simulink model "rev0BB"  (R2014b)
settings: Solver=FixedStepDiscrete  SolverMode=SingleTasking  StartTime=0  StopTime=12000*basePer  RelTol=1e-3
StartFcn:
  | clc;
StopFcn:
  | disp('');
values from neighbouring files (symbols this model uses):
  baseFreq = overSampleFreq/overSample    (= 62.5)    [rev0BB_setup.m]    (also in rev0BB_startup.m = 31.25)
  basePer = 1/baseFreq    (= 0.016)    [rev0BB_setup.m]    (also in rev0BB_startup.m = 0.032)
  cbTol = int16(5)    [rev0BB_setup.m]    (also in rev0BB_startup.m)
  cef_note_len = uint16(length(cef_note))    [rev0BB_setup.m]    (also in rev0BB_startup.m)
  cr_int_amp = 2^-4    (= 0.0625)    [rev0BB_setup.m]
  cr_int_preamp = 2^-8    (= 0.00390625)    [rev0BB_setup.m]
  cr_pre_amp = 1    [rev0BB_setup.m]
  cr_smooth_amp = 2^-4    (= 0.0625)    [rev0BB_setup.m]
  cr_smooth_num = (1/cr_smooth_samples).*ones(1, cr_smooth_samples)    [rev0BB_setup.m]
  cr_smooth_second_denom = [1, -0.30]    [rev0BB_setup.m]
  D_128 = [ 1,  8,  2,  4, 16, 32, 64]    [golay.m]    (also in rev0BB_setup.m; rev0BB_startup.m = D_128 .* 4)
  dataDelay = length(cat(1, xCTRL_PRE_adj, guard, startWord)) + 1 + 187    [rev0BB_setup.m]    (also in rev0BB_startup.m = length(cat(1, xCTRL_PRE_adj, guard, startWord)) + 1)
  dataLen = 4096    [rev0BB_setup.m]    (also in rev0BB_startup.m)
  expDomain = 3.3    [rev0BB_setup.m]    (also in rev0BB_startup.m)
  expectedPer = int16(128*expectedWidth)    [rev0BB_setup.m]    (also in rev0BB_startup.m)
  expectedWidth = int16(1)    [rev0BB_setup.m]    (also in rev0BB_startup.m = int16(4))
  expResolution = 2^-7    (= 0.0078125)    [rev0BB_setup.m]    (also in rev0BB_startup.m)
  expTol = .1    (= 0.1)    [rev0BB_setup.m]    (also in rev0BB_startup.m)
  freqOffsetFactor = 0.001    [rev0BB_setup.m]
  guardInt = int16(4)    [rev0BB_setup.m]    (also in rev0BB_startup.m)
  guardTol = int16(5)    [rev0BB_setup.m]    (also in rev0BB_startup.m)
  invertedTol = int16(8)    [rev0BB_setup.m]    (also in rev0BB_startup.m)
  lineWidth = 60    [rev0BB_setup.m]    (also in rev0BB_startup.m)
  mult_pipeline = 3    [rev0BB_setup.m]
  overSamplePer = 1/overSampleFreq    (= 0.004)    [rev0BB_setup.m]    (also in rev0BB_startup.m = 0.008)
  rcRxFilt = [0.0136862302916632 -1.07255950749522e-17 -0.0189771276893529 -0.0291239876115654 -0.0188755211158258 0.0106361356824736 0.0424635782726055 0.0519988855587596 0.023305426798367 -0.0360582703762239 -0.092415015279578 -0.100052449159764 -0.0262868760771072 0.126203946316784 0.313718534732932 0.467989970028836 0.527600531456874 0.467989970028836 0.313718534732932 0.126203946316784 -0.0262868760771072 ...(+235 chars)    [rev0BB_setup.m]
  regular_pipeline = 1    [rev0BB_setup.m]
  smooth_num = (1).*(1/smooth_samples).*ones(1, smooth_samples)    [rev0BB_setup.m]
  smooth_scale = 0.0003    [rev0BB_setup.m]
  smooth_second_denom = [1, -0.95]    [rev0BB_setup.m]
  tol = int16(15)    [rev0BB_setup.m]    (also in rev0BB_startup.m)
  trigger = 60    [rev0BB_setup.m]    (also in rev0BB_startup.m)
  W_128 = [-1, -1, -1, -1, +1, -1, -1]    [golay.m]    (also in rev0BB_setup.m; rev0BB_startup.m)
  wordLen = int16(8)    [rev0BB_setup.m]    (also in rev0BB_startup.m)
undefined symbols (not defined in the file or in its folder): i, idealX
libraries: helperLib x11, golayLib x7, simulink x5, commdigbbndpm3 x4, dsparch4 x2, dspmlti4 x2, commfilt2 x2, commchan3 x1, commsink2 x1, commrflib2 x1, dspsigops x1, hdlsllib x1
settings Model: FPTRunName=FPA_Reference  Creator=cyarp  LastModifiedBy=cyarp
settings DataIOCC: SaveOutput=off  SignalLogging=off  SaveTime=off
settings OptimizationCC: BlockReduction=off  ConditionallyExecuteInputs=off  InlineParams=on  SimCompilerOptimization=On
settings DebuggingCC: AlgebraicLoopMsg=error  SingleTaskRateTransMsg=error
settings HardwareCC: ProdHWDeviceType=ASIC/FPGA->ASIC/FPGA  TargetBitPerLong=64  TargetBitPerPointer=64  TargetLongLongMode=on  TargetIntDivRoundTo=Zero  TargetEndianess=LittleEndian  TargetWordSize=64  TargetHWDeviceType=MATLAB Host  ProdEqTarget=off

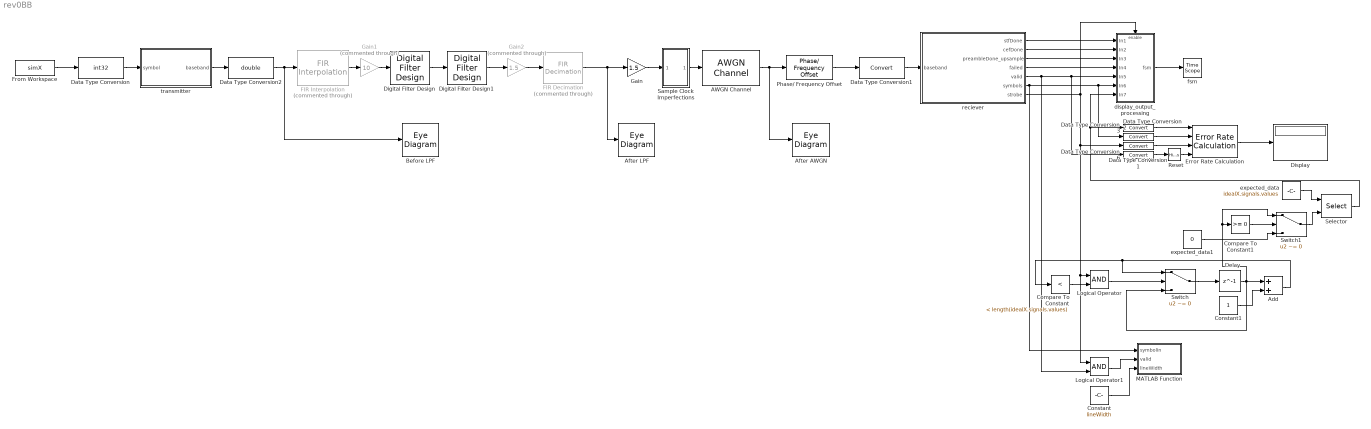
== system rev0BB ==
  AWGN Channel : commchan3/AWGN Channel  InputProcessing=Columns as channels (frame based)  seed=67  noiseMode="Signal to noise ratio  (Eb/No)"  EbNodB=awgnEbN0  EsNodB=10  SNRdB=10  bitsPerSym=1  Ps=1  Tsym=basePer*4  variance=1
  Add : Sum
  After AWGN : EyeDiagram
  After LPF : EyeDiagram
  Before LPF : EyeDiagram
  Compare To Constant : simulink/Logic and Bit Operations/Compare To Constant  relop=<  const=length(idealX.signals.values)  OutDataTypeStr=boolean
  Compare To Constant1 : simulink/Logic and Bit Operations/Compare To Constant  relop=>=  const=0  OutDataTypeStr=boolean
  Constant : Constant  Value=lineWidth
  Constant1 : Constant
  Data Type Conversion{1,1..3,6} (5 alike) : DataTypeConversion
  Data Type Conversion : DataTypeConversion  OutDataTypeStr=int32  RndMeth=Nearest
  Data Type Conversion2 : DataTypeConversion  OutDataTypeStr=double  RndMeth=Nearest
  Delay : Delay  DelayLength=1  InitialCondition=-dataDelay
  Digital Filter Design : dsparch4/Digital Filter Design  mwdsp_browser_bugfix_var=off
  Digital Filter Design1 : dsparch4/Digital Filter Design  mwdsp_browser_bugfix_var=off
  Display : Display
  Error Rate Calculation : commsink2/Error Rate Calculation  N=0  st_delay=0  cp_mode=Select samples from port  subframe=[]  PMode=Port  WsName=ErrorVec  RsMode2=on  stop=off  numErr=100  maxBits=1e6
  FIR Decimation : dspmlti4/FIR Decimation  Commented=through  h=fir1(35,0.4)  D=16  filtStruct=Direct form  framing=Enforce single-rate processing  inputOffset=0  outputBufInitCond=0  InputProcessing=Columns as channels (frame based)  firstCoeffDataTypeStr=Inherit: Same word length as input  firstCoeffLastDataTypeStr=Inherit: Same word length as input  firstCoeffMin=[]  firstCoeffMax=[]  outputDataTypeStr=Inherit: Same as accumulator  outputLastDataTypeStr=Inherit: Same as accumulator  outputMin=[]  outputMax=[]  roundingMode=Floor  overflowMode=off  FilterSource=Specify via dialog  FilterObject=Hm_firdecim
      settings: allowOverrides=off
  FIR Interpolation : dspmlti4/FIR Interpolation  Commented=through  h=fir1(15,1/4)  L=16  framing=Enforce single-rate processing  outputBufInitCond=0  InputProcessing=Columns as channels (frame based)  firstCoeffDataTypeStr=Inherit: Same word length as input  firstCoeffLastDataTypeStr=Inherit: Same word length as input  firstCoeffMin=[]  firstCoeffMax=[]  outputDataTypeStr=Inherit: Same as accumulator  outputLastDataTypeStr=Inherit: Same as accumulator  outputMin=[]  outputMax=[]  roundingMode=Floor  overflowMode=off  FilterSource=Specify via dialog  FilterObject=Hm_firinterp
  From Workspace : FromWorkspace  VariableName=simX  SampleTime=basePer*1  Interpolate=off  OutputAfterFinalValue=Setting to zero
  Gain : Gain  Gain=1.5
  Gain1 : Gain  Commented=through  Gain=10
  Gain2 : Gain  Commented=through  Gain=1.5
  Logical Operator : Logic  AllPortsSameDT=off  OutDataTypeStr=boolean
  Logical Operator1 : Logic  AllPortsSameDT=off  OutDataTypeStr=boolean
  MATLAB Function : MATLAB Function  TreatAsAtomicUnit=on
  Phase/ Frequency Offset : commrflib2/Phase// Frequency Offset  phaseOffset=180  freqPort=off  freqOffset=freqOffsetFactor*baseFreq
  Reset : HitCross  HitCrossingOffset=0.5  HitCrossingDirection=rising
  Sample Clock Imperfections : Subsystem
  Selector : Selector  IndexMode=Zero-based  InputPortWidth=length(idealX.signals.values)  IndexOptions=Index vector (port)  Indices=[1 3]
  Switch : Switch  Criteria=u2 ~= 0
  Switch1 : Switch  Criteria=u2 ~= 0
  display_output_processing : Subsystem
  expected_data : Constant  Value=idealX.signals.values
  expected_data1 : Constant  Value=0
  fsm : TimeScope  DefaultConfigurationName=spbscopes.TimeScopeBlockCfg
  reciever : Subsystem
  transmitter : Subsystem
  wires:
  Data Type Conversion1/1 -> reciever/1(baseband)
  Data Type Conversion/1 -> transmitter/1(symbol)
  transmitter/1(baseband) -> Data Type Conversion2/1
  From Workspace/1 -> Data Type Conversion/1
  Digital Filter Design1/1 -> Gain2/1
  Gain/1 -> Sample Clock Imperfections/1(In1)
  Digital Filter Design/1 -> Digital Filter Design1/1
  Sample Clock Imperfections/1(Out1) -> AWGN Channel/1
  AWGN Channel/1 -> After AWGN/1, Phase/ Frequency Offset/1
  Phase/ Frequency Offset/1 -> Data Type Conversion1/1
  reciever/1(stfDone) -> display_output_processing/1(In1)
  reciever/2(cefDone) -> display_output_processing/2(In2)
  reciever/3(preambleDone_upsample) -> display_output_processing/3(In3)
  reciever/4(failed) -> display_output_processing/4(In4)
  reciever/5(valid) -> Logical Operator1/2, Data Type Conversion6/1, display_output_processing/5(In5)
  Selector/1 -> Data Type Conversion3/1, display_output_processing/7(In7)
  display_output_processing/1(fsm) -> fsm/1
  Error Rate Calculation/1 -> Display/1
  Data Type Conversion6/1 -> Reset/1
  Reset/1 -> Error Rate Calculation/4
  Data Type Conversion1/1 -> Error Rate Calculation/3
  Data Type Conversion2/1 -> Error Rate Calculation/2
  Data Type Conversion3/1 -> Error Rate Calculation/1
  expected_data/1 -> Selector/1
  Constant1/1 -> Add/2
  Add/1 -> Switch/1, Compare To Constant/1
  Switch/1 -> Delay/1
  Compare To Constant/1 -> Logical Operator/2
  Logical Operator/1 -> Switch/2
  Delay/1 -> Switch1/1, Compare To Constant1/1, Switch/3, Add/1
  Switch1/1 -> Selector/2
  Compare To Constant1/1 -> Switch1/2
  expected_data1/1 -> Switch1/3
  reciever/7(strobe) -> display_output_processing/Enable, Logical Operator1/1, Logical Operator/1, Data Type Conversion1/1
  reciever/6(symbols) -> MATLAB Function/1(symbolIn), display_output_processing/6(In6), Data Type Conversion2/1
  Constant/1 -> MATLAB Function/3(lineWidth)
  Logical Operator1/1 -> MATLAB Function/2(valid)
  FIR Interpolation/1 -> Gain1/1
  Data Type Conversion2/1 -> FIR Interpolation/1, Before LPF/1
  Gain1/1 -> Digital Filter Design/1
  FIR Decimation/1 -> After LPF/1, Gain/1
  Gain2/1 -> FIR Decimation/1

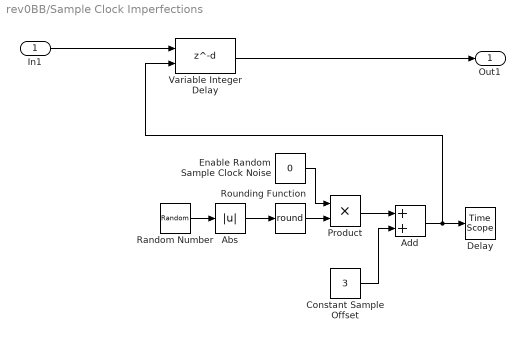
== system rev0BB/Sample Clock Imperfections ==
  In1 : Inport
  Abs : Abs
  Add : Sum
  Constant Sample Offset : Constant  Value=3
  Delay : TimeScope  DefaultConfigurationName=spbscopes.TimeScopeBlockCfg
  Enable Random Sample Clock Noise : Constant  Value=0
  Product : Product
  Random Number : RandomNumber  Variance=.5  SampleTime=overSamplePer
  Rounding Function : Rounding  Operator=round
  Variable Integer Delay : Delay  DelayLengthSource=Input port
      settings: InputPortMap=u0,p1
  Out1 : Outport
  wires:
  Abs/1 -> Rounding Function/1
  Random Number/1 -> Abs/1
  Add/1 -> Delay/1, Variable Integer Delay/2
  Enable Random Sample Clock Noise/1 -> Product/1
  Constant Sample Offset/1 -> Add/2
  Rounding Function/1 -> Product/2
  Product/1 -> Add/1
  In1/1 -> Variable Integer Delay/1
  Variable Integer Delay/1 -> Out1/1

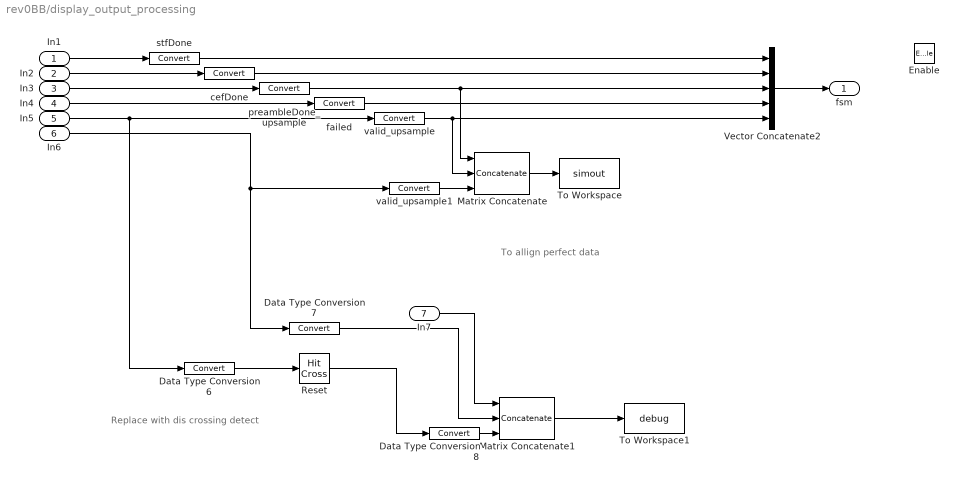
== system rev0BB/display_output_processing ==
  note: To allign perfect data
  note: Replace with dis crossing detect
  In1 : Inport
  In2 : Inport  Port=2
  In3 : Inport  Port=3
  In4 : Inport  Port=4
  In5 : Inport  Port=5
  In6 : Inport  Port=6
  In7 : Inport  Port=7
  Enable : EnablePort
  Data Type Conversion6 : DataTypeConversion
  Data Type Conversion7 : DataTypeConversion
  Data Type Conversion8 : DataTypeConversion
  Matrix Concatenate : Concatenate  NumInputs=3  Mode=Multidimensional array  ConcatenateDimension=2
  Matrix Concatenate1 : Concatenate  NumInputs=3  Mode=Multidimensional array  ConcatenateDimension=2
  Reset : HitCross  HitCrossingOffset=0.5  HitCrossingDirection=rising
  To Workspace : ToWorkspace  VariableName=simout  SampleTime=-1
      settings: Save2DSignal=2-D array (concatenate along first dimension)
  To Workspace1 : ToWorkspace  VariableName=debug  SampleTime=-1
      settings: Save2DSignal=2-D array (concatenate along first dimension)
  Vector Concatenate2 : Concatenate  NumInputs=5  Mode=Multidimensional array  ConcatenateDimension=2
  cefDone : DataTypeConversion
  failed : DataTypeConversion
  preambleDone_upsample : DataTypeConversion
  stfDone : DataTypeConversion
  valid_upsample : DataTypeConversion
  valid_upsample1 : DataTypeConversion
  fsm : Outport
  wires:
  Vector Concatenate2/1 -> fsm/1
  Matrix Concatenate/1 -> To Workspace/1
  stfDone/1 -> Vector Concatenate2/1
  cefDone/1 -> Vector Concatenate2/2
  preambleDone_upsample/1 -> Matrix Concatenate/1, Vector Concatenate2/3
  failed/1 -> Vector Concatenate2/4
  Data Type Conversion6/1 -> Reset/1
  In7/1 -> Matrix Concatenate1/1
  Matrix Concatenate1/1 -> To Workspace1/1
  Data Type Conversion8/1 -> Matrix Concatenate1/3
  Data Type Conversion7/1 -> Matrix Concatenate1/2
  Reset/1 -> Data Type Conversion8/1
  In1/1 -> stfDone/1
  In2/1 -> cefDone/1
  In3/1 -> preambleDone_upsample/1
  In4/1 -> failed/1
  valid_upsample/1 -> Matrix Concatenate/2, Vector Concatenate2/5
  valid_upsample1/1 -> Matrix Concatenate/3
  In5/1 -> Data Type Conversion6/1, valid_upsample/1
  In6/1 -> Data Type Conversion7/1, valid_upsample1/1

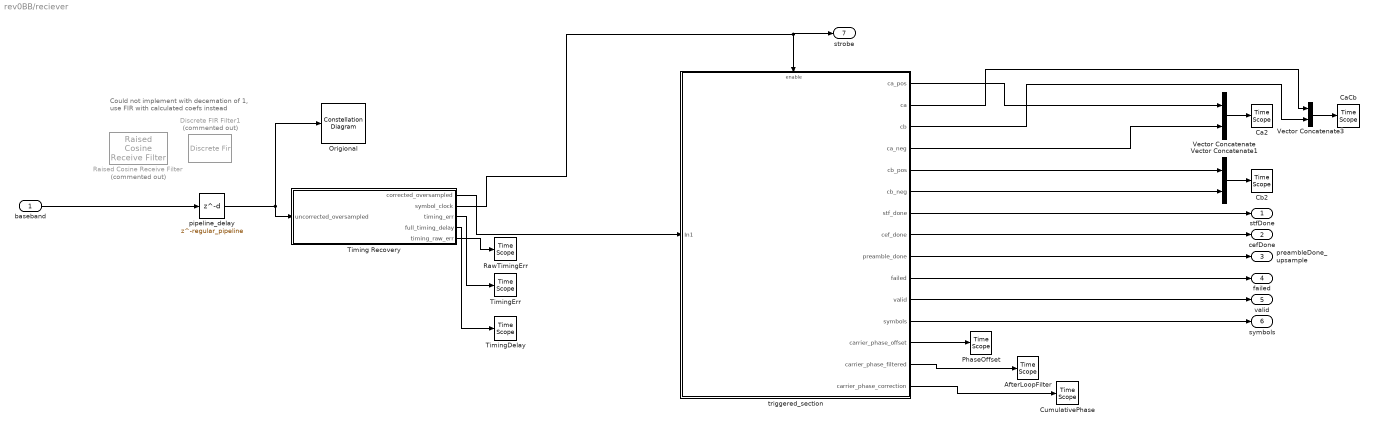
== system rev0BB/reciever ==
  note: Could not implement with decemation
      | of 1, use FIR with calculated coefs instead
  baseband : Inport  OutDataTypeStr=fixdt(1,14,11)  SampleTime=overSamplePer
  AfterLoopFilter : TimeScope  DefaultConfigurationName=spbscopes.TimeScopeBlockCfg
  Ca2 : TimeScope  DefaultConfigurationName=spbscopes.TimeScopeBlockCfg
  CaCb : TimeScope  DefaultConfigurationName=spbscopes.TimeScopeBlockCfg
  Cb2 : TimeScope  DefaultConfigurationName=spbscopes.TimeScopeBlockCfg
  CumulativePhase : TimeScope  DefaultConfigurationName=spbscopes.TimeScopeBlockCfg
  Discrete FIR Filter1 : DiscreteFir  Commented=on  Coefficients=rcRxFilt
  Origional : ConstellationDiagram
  PhaseOffset : TimeScope  DefaultConfigurationName=spbscopes.TimeScopeBlockCfg
  Raised Cosine Receive Filter : commfilt2/Raised Cosine Receive Filter  Commented=on  filtType=Normal  N=4  filtSpan=16  currentFiltSpan=16  D=(16)/2  R=.2  sampMode=Mute  saveAsFlag=0  rateMode=Downsampling  downFactor=1  downOffset=0  framing=Allow multirate processing  checkGain=Normalized  filterGain=1  checkCoeff=on  variableName=rcRxFilt  launchFVT=on  roundingMode=Floor  overflowMode=off
  RawTimingErr : TimeScope  DefaultConfigurationName=spbscopes.TimeScopeBlockCfg
  Timing Recovery : Subsystem
  TimingDelay : TimeScope  DefaultConfigurationName=spbscopes.TimeScopeBlockCfg
  TimingErr : TimeScope  DefaultConfigurationName=spbscopes.TimeScopeBlockCfg
  Vector Concatenate : Concatenate  Mode=Multidimensional array  ConcatenateDimension=2
  Vector Concatenate1 : Concatenate  Mode=Multidimensional array  ConcatenateDimension=2
  Vector Concatenate3 : Concatenate  Mode=Multidimensional array  ConcatenateDimension=2
  pipeline_delay : Delay  DelayLength=regular_pipeline
  triggered_section : Subsystem
  stfDone : Outport
  cefDone : Outport  Port=2
  preambleDone_upsample : Outport  Port=3
  failed : Outport  Port=4
  valid : Outport  Port=5
  symbols : Outport  Port=6
  strobe : Outport  Port=7
  wires:
  Vector Concatenate/1 -> Ca2/1
  Vector Concatenate1/1 -> Cb2/1
  Vector Concatenate3/1 -> CaCb/1
  Timing Recovery/2(symbol_clock) -> triggered_section/Enable, strobe/1
  triggered_section/1(ca_pos) -> Vector Concatenate/1
  triggered_section/2(ca) -> Vector Concatenate3/1
  triggered_section/3(cb) -> Vector Concatenate3/2
  triggered_section/4(ca_neg) -> Vector Concatenate/2
  triggered_section/5(cb_pos) -> Vector Concatenate1/1
  triggered_section/6(cb_neg) -> Vector Concatenate1/2
  triggered_section/7(stf_done) -> stfDone/1
  triggered_section/8(cef_done) -> cefDone/1
  triggered_section/9(preamble_done) -> preambleDone_upsample/1
  triggered_section/10(failed) -> failed/1
  triggered_section/11(valid) -> valid/1
  triggered_section/12(symbols) -> symbols/1
  Timing Recovery/1(corrected_oversampled) -> triggered_section/1(In1)
  pipeline_delay/1 -> Origional/1, Timing Recovery/1(uncorrected_oversampled)
  baseband/1 -> pipeline_delay/1
  triggered_section/13(carrier_phase_offset) -> PhaseOffset/1
  triggered_section/14(carrier_phase_filtered) -> AfterLoopFilter/1
  triggered_section/15(carrier_phase_correction) -> CumulativePhase/1
  Timing Recovery/3(timing_err) -> TimingErr/1
  Timing Recovery/4(full_timing_delay) -> TimingDelay/1
  Timing Recovery/5(timing_raw_err) -> RawTimingErr/1

== system rev0BB/transmitter ==
  symbol : Inport
  BPSK Modulator Baseband : commdigbbndpm3/BPSK Modulator Baseband  Ph=0  outDtype=Fixed-point  outWordLen=16  outUDDataType=sfix(16)  outFracLenMode=User-defined  outFracLen=11
  Raised Cosine Transmit Filter : commfilt2/Raised Cosine Transmit Filter  filtType=Normal  filtSpan=16  currentFiltSpan=16  D=(16)/2  R=0.2  sampMode=Mute  saveAsFlag=0  N=4  framing=Allow multirate processing  checkGain=Normalized  filterGain=1  checkCoeff=off  variableName=rcTxFilt  launchFVT=on  roundingMode=Floor  overflowMode=off
  baseband : Outport
  wires:
  symbol/1 -> BPSK Modulator Baseband/1
  BPSK Modulator Baseband/1 -> Raised Cosine Transmit Filter/1
  Raised Cosine Transmit Filter/1 -> baseband/1

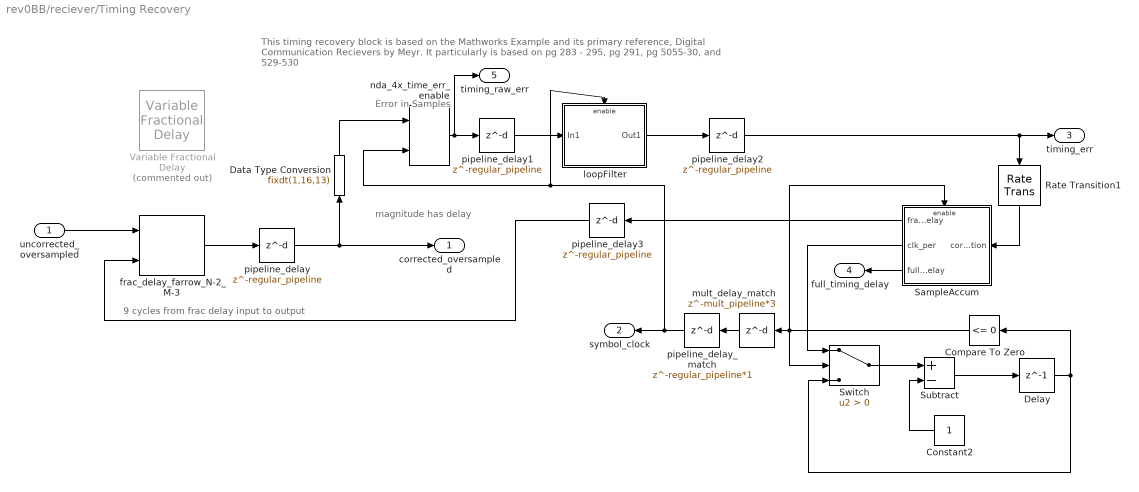
== system rev0BB/reciever/Timing Recovery ==
  note: 9 cycles from frac delay input to output
  note: Error in Samples
  note: magnitude has delay
  note: This timing recovery block is based on the Mathworks Example and its primary reference, Digital Communication Recievers by Meyr. It particularly is based on pg 283 - 295, pg 291, pg 5055-30, and 529-530
  uncorrected_oversampled : Inport
  Compare To Zero : simulink/Logic and Bit Operations/Compare To Zero  relop=<=  OutDataTypeStr=boolean
  Constant2 : Constant  OutDataTypeStr=Inherit: Inherit via back propagation
  Data Type Conversion : DataTypeConversion  OutDataTypeStr=fixdt(1,16,13)
  Delay : Delay  DelayLength=1  InitialCondition=0
  Rate Transition1 : RateTransition
  SampleAccum : Subsystem
  Subtract : Sum  Inputs=+-
  Switch : Switch  Criteria=u2 > Threshold
  Variable Fractional Delay : dspsigops/Variable Fractional Delay  Commented=on  mode=OBSOLETE  modeActive=Linear  dmax=1  L=4  FarrowL=2  R=10  alpha=1  ic=0  fallbackFIR=Clip to the minimum value necessary for centered kernel  fallbackFarrow=Clip to the minimum value necessary for centered kernel  noDFT=off  roundingMode=Zero  overflowMode=off
  frac_delay_farrow_N-2_M-3 : helperLib/frac_delay_farrow_N-2_M-3
  loopFilter : Subsystem
  mult_delay_match : Delay  DelayLength=mult_pipeline*3
  nda_4x_time_err_enable : helperLib/nda_4x_time_err_enable
      link override phase_est/timing_rec_sym_rate_enb/atan2/inv Lookup Table: OutDataTypeStr=fixdt(1,16,2)  Table=[(1./(-8:frac_lut_res:(0-frac_lut_res))), 1/frac_lut_res, (1./((0+frac_lut_res):frac_lut_res:7))]  RemoveProtectionInput=off  BreakpointsForDimension1=-8:frac_lut_res:7
  pipeline_delay{,1..3} (4 alike) : Delay  DelayLength=regular_pipeline
  pipeline_delay_match : Delay  DelayLength=regular_pipeline*1
  corrected_oversampled : Outport
  symbol_clock : Outport  Port=2
  timing_err : Outport  Port=3
  full_timing_delay : Outport  Port=4
  timing_raw_err : Outport  Port=5
  wires:
  Delay/1 -> Compare To Zero/1, Switch/3
  Switch/1 -> Subtract/1
  Constant2/1 -> Subtract/2
  Rate Transition1/1 -> SampleAccum/1(correction)
  nda_4x_time_err_enable/1 -> timing_raw_err/1, pipeline_delay1/1
  SampleAccum/2(clk_per) -> Switch/1
  Subtract/1 -> Delay/1
  loopFilter/1(Out1) -> pipeline_delay2/1
  pipeline_delay1/1 -> loopFilter/1(In1)
  uncorrected_oversampled/1 -> frac_delay_farrow_N-2_M-3/1
  SampleAccum/3(fullDelay) -> full_timing_delay/1
  pipeline_delay2/1 -> Rate Transition1/1, timing_err/1
  SampleAccum/1(fracDelay) -> pipeline_delay3/1
  Compare To Zero/1 -> SampleAccum/Enable, mult_delay_match/1, Switch/2
  mult_delay_match/1 -> pipeline_delay_match/1
  frac_delay_farrow_N-2_M-3/1 -> pipeline_delay/1
  pipeline_delay_match/1 -> symbol_clock/1, nda_4x_time_err_enable/2, loopFilter/Enable
  pipeline_delay3/1 -> frac_delay_farrow_N-2_M-3/2
  pipeline_delay/1 -> Data Type Conversion/1, corrected_oversampled/1
  Data Type Conversion/1 -> nda_4x_time_err_enable/1

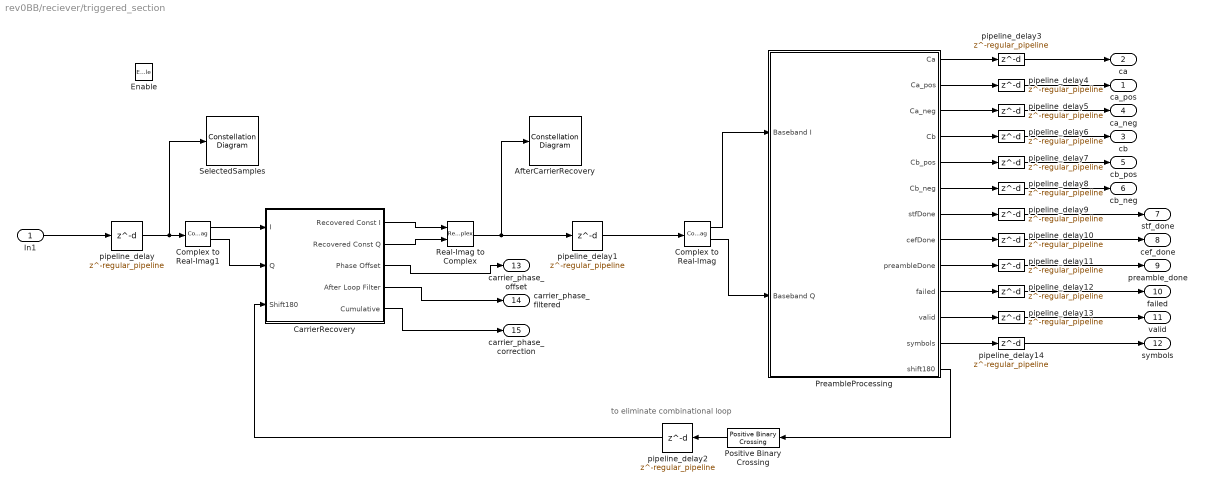
== system rev0BB/reciever/triggered_section ==
  note: to eliminate combinational loop
  In1 : Inport
  Enable : EnablePort
  " AfterCarrierRecovery" : ConstellationDiagram
  " SelectedSamples" : ConstellationDiagram
  CarrierRecovery : Subsystem  RequirementInfo={'linktype_rmi_matlab' 'rev0BB_startup' '@736102.1' 'true' 'loop' '' } %GIDa_d02aedaf_4fff_4ad7_becd_06d8542c600d
  Complex to Real-Imag : ComplexToRealImag
  Complex to Real-Imag1 : ComplexToRealImag
  Positive Binary Crossing : helperLib/Positive Binary Crossing
  PreambleProcessing : Subsystem  TreatAsAtomicUnit=on
  Real-Imag to Complex : RealImagToComplex
  pipeline_delay{,1..14} (15 alike) : Delay  DelayLength=regular_pipeline
  ca_pos : Outport  InitialOutput=0
  ca : Outport  Port=2  InitialOutput=0
  cb : Outport  Port=3  InitialOutput=0
  ca_neg : Outport  Port=4  InitialOutput=0
  cb_pos : Outport  Port=5  InitialOutput=0
  cb_neg : Outport  Port=6  InitialOutput=0
  stf_done : Outport  Port=7  InitialOutput=0
  cef_done : Outport  Port=8  InitialOutput=0
  preamble_done : Outport  Port=9  InitialOutput=0
  failed : Outport  Port=10  InitialOutput=0
  valid : Outport  Port=11  InitialOutput=0
  symbols : Outport  Port=12  InitialOutput=0
  carrier_phase_offset : Outport  Port=13  InitialOutput=0
  carrier_phase_filtered : Outport  Port=14  InitialOutput=0
  carrier_phase_correction : Outport  Port=15  InitialOutput=0
  wires:
  pipeline_delay1/1 -> Complex to Real-Imag/1
  PreambleProcessing/7(stfDone) -> pipeline_delay9/1
  PreambleProcessing/8(cefDone) -> pipeline_delay10/1
  PreambleProcessing/9(preambleDone) -> pipeline_delay11/1
  PreambleProcessing/10(failed) -> pipeline_delay12/1
  PreambleProcessing/11(valid) -> pipeline_delay13/1
  Complex to Real-Imag/1 -> PreambleProcessing/1(Baseband I)
  Complex to Real-Imag/2 -> PreambleProcessing/2(Baseband Q)
  Complex to Real-Imag1/1 -> CarrierRecovery/1(I)
  Complex to Real-Imag1/2 -> CarrierRecovery/2(Q)
  CarrierRecovery/1(Recovered Const I) -> Real-Imag to Complex/1
  CarrierRecovery/2(Recovered Const Q) -> Real-Imag to Complex/2
  CarrierRecovery/3(Phase Offset) -> carrier_phase_offset/1
  CarrierRecovery/4(After Loop Filter) -> carrier_phase_filtered/1
  CarrierRecovery/5(Cumulative) -> carrier_phase_correction/1
  pipeline_delay2/1 -> CarrierRecovery/3(Shift180)
  PreambleProcessing/12(symbols) -> pipeline_delay14/1
  PreambleProcessing/1(Ca) -> pipeline_delay3/1
  PreambleProcessing/2(Ca_pos) -> pipeline_delay4/1
  PreambleProcessing/3(Ca_neg) -> pipeline_delay5/1
  PreambleProcessing/4(Cb) -> pipeline_delay6/1
  PreambleProcessing/5(Cb_pos) -> pipeline_delay7/1
  PreambleProcessing/6(Cb_neg) -> pipeline_delay8/1
  pipeline_delay/1 -> " SelectedSamples"/1, Complex to Real-Imag1/1
  pipeline_delay14/1 -> symbols/1
  pipeline_delay13/1 -> valid/1
  pipeline_delay12/1 -> failed/1
  pipeline_delay11/1 -> preamble_done/1
  pipeline_delay10/1 -> cef_done/1
  pipeline_delay9/1 -> stf_done/1
  pipeline_delay8/1 -> cb_neg/1
  pipeline_delay7/1 -> cb_pos/1
  pipeline_delay6/1 -> cb/1
  pipeline_delay5/1 -> ca_neg/1
  pipeline_delay4/1 -> ca_pos/1
  pipeline_delay3/1 -> ca/1
  Positive Binary Crossing/1 -> pipeline_delay2/1
  Real-Imag to Complex/1 -> pipeline_delay1/1, " AfterCarrierRecovery"/1
  In1/1 -> pipeline_delay/1
  PreambleProcessing/13(shift180) -> Positive Binary Crossing/1

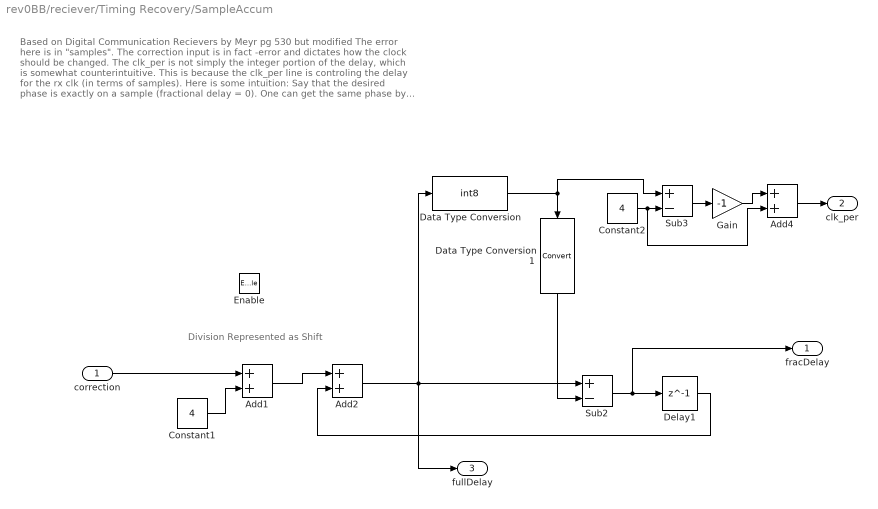
== system rev0BB/reciever/Timing Recovery/SampleAccum ==
  note: Division Represented as Shift
  note: Based on Digital Communication Recievers by Meyr pg 530 but modified
      |
      | The error here is in "samples". The correction input is in fact -error and
      | dictates how the clock should be changed.
      |
      | The clk_per is not simply the integer portion of the delay, which is
      | somewhat counterintuitive. This is because the clk_per line is controling
      | the delay for the rx clk (in terms of samples). Here is some intuition:
      | Say that the desired phase is exactly on a sample (fractional delay = 0).
      | One can get the same phase by setting the fractional phase to 1 but the
      | clock must add 1 sample to catch up with the additional delay added.
      |
      | The same logic holds true in the reverse case. Delay can be changed
      | from 1 to 0 but the clock must skip a sample to catch up.
      |
      | Diagrams showing the clock logic as well as the logic when a phase correction
      | is non-zeros are presented to the left of this text.
  correction : Inport
  Enable : EnablePort
  Add1 : Sum  OutDataTypeStr=Inherit: Same as first input
  Add2 : Sum  OutDataTypeStr=Inherit: Same as first input
  Add4 : Sum  OutDataTypeStr=Inherit: Same as first input
  Constant1 : Constant  Value=4  OutDataTypeStr=Inherit: Inherit via back propagation
  Constant2 : Constant  Value=4  OutDataTypeStr=Inherit: Inherit via back propagation
  Data Type Conversion : DataTypeConversion  OutDataTypeStr=int8
  Data Type Conversion1 : DataTypeConversion
  Delay1 : Delay  DelayLength=1  InitialCondition=0
  Gain : Gain  Gain=-1  OutDataTypeStr=Inherit: Same as input
  Sub2 : Sum  Inputs=+-  OutDataTypeStr=Inherit: Same as first input
  Sub3 : Sum  Inputs=+-  OutDataTypeStr=Inherit: Same as first input
  fracDelay : Outport  InitialOutput=[0]
  clk_per : Outport  Port=2  InitialOutput=[0]
  fullDelay : Outport  Port=3  InitialOutput=[0]
  wires:
  Add2/1 -> fullDelay/1, Sub2/1, Data Type Conversion/1
  Sub2/1 -> fracDelay/1, Delay1/1
  Data Type Conversion1/1 -> Sub2/2
  Data Type Conversion/1 -> Sub3/1, Data Type Conversion1/1
  Delay1/1 -> Add2/2
  correction/1 -> Add1/1
  Constant1/1 -> Add1/2
  Add1/1 -> Add2/1
  Constant2/1 -> Add4/2, Sub3/2
  Sub3/1 -> Gain/1
  Gain/1 -> Add4/1
  Add4/1 -> clk_per/1

== system rev0BB/reciever/Timing Recovery/loopFilter ==
  In1 : Inport
  Enable : EnablePort
  Add : Sum
  Discrete FIR Filter : DiscreteFir  FilterStructure=Direct form symmetric  Coefficients=smooth_num  OutDataTypeStr=Inherit: Same as input
  Gain : Gain  Gain=smooth_scale  OutDataTypeStr=Inherit: Same as input
  cr_smooth_int : Gain  Gain=-smooth_second_denom(2)  OutDataTypeStr=Inherit: Same as input
  mult_delay1 : Delay  DelayLength=mult_pipeline
  mult_delay2 : Delay  DelayLength=mult_pipeline
  mult_delay4 : Delay  DelayLength=mult_pipeline
  Out1 : Outport  InitialOutput=0
  wires:
  Gain/1 -> mult_delay4/1
  mult_delay1/1 -> Gain/1, Add/2
  mult_delay4/1 -> Out1/1
  In1/1 -> Discrete FIR Filter/1
  Discrete FIR Filter/1 -> mult_delay2/1
  Add/1 -> cr_smooth_int/1
  cr_smooth_int/1 -> mult_delay1/1
  mult_delay2/1 -> Add/1

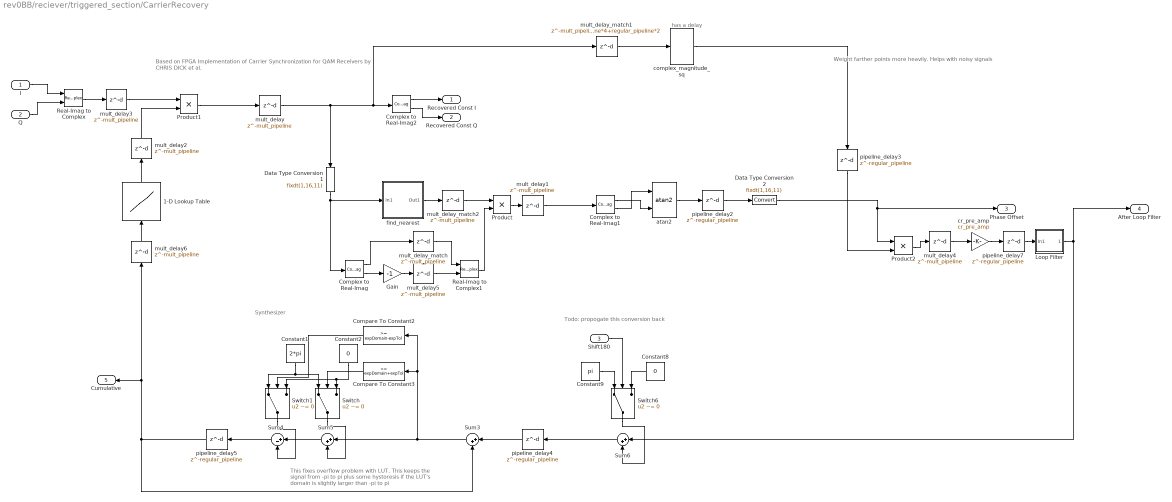
== system rev0BB/reciever/triggered_section/CarrierRecovery ==
  note: Weight farther points more heavily. Helps with noisy signals
  note: has a delay
  note: Synthesizer
  note: Todo: propogate this conversion back
  note: This fixes overflow problem with LUT.  This keeps the
      | signal from -pi to pi plus some hystoresis if the LUT's
      | domain is slightly larger than -pi to pi
  note: Based on FPGA Implementation of Carrier Synchronization for QAM Receivers
      | by CHRIS DICK et al.
  I : Inport  OutDataTypeStr=fixdt(1,14,11)  PortDimensions=1  SampleTime=overSamplePer
  Q : Inport  Port=2  OutDataTypeStr=fixdt(1,14,11)  PortDimensions=1  SampleTime=overSamplePer
  Shift180 : Inport  Port=3  OutDataTypeStr=boolean  PortDimensions=1  SampleTime=overSamplePer
  1-D Lookup Table : Lookup_n-D  NumberOfTableDimensions=1  BreakpointsForDimension1=[-expDomain:expResolution:expDomain]  IndexSearchMethod=Evenly spaced points  Table=exp(i*[-expDomain:expResolution:expDomain])  InterpMethod=Flat  DiagnosticForOutOfRangeInput=Error  InternalRulePriority=Speed  RndMeth=Simplest  InputSameDT=on
  Compare To Constant2 : simulink/Logic and Bit Operations/Compare To Constant  relop=>=  const=expDomain-expTol  OutDataTypeStr=boolean
  Compare To Constant3 : simulink/Logic and Bit Operations/Compare To Constant  relop=<=  const=-expDomain+expTol  OutDataTypeStr=boolean
  Complex to Real-Imag : ComplexToRealImag
  Complex to Real-Imag1 : ComplexToRealImag
  Complex to Real-Imag2 : ComplexToRealImag
  Constant1 : Constant  Value=2*pi  OutDataTypeStr=Inherit: Inherit via back propagation
  Constant2 : Constant  Value=0  OutDataTypeStr=Inherit: Inherit via back propagation
  Constant8 : Constant  Value=0  OutDataTypeStr=fixdt(1,16,11)
  Constant9 : Constant  Value=pi  OutDataTypeStr=fixdt(1,16,11)
  Data Type Conversion1 : DataTypeConversion  OutDataTypeStr=fixdt(1,16,11)
  Data Type Conversion2 : DataTypeConversion  OutDataTypeStr=fixdt(1,16,11)
  Gain : Gain  Gain=-1  OutDataTypeStr=Inherit: Same as input
  Loop Filter : Subsystem
  Product : Product  OutDataTypeStr=Inherit: Same as first input
  Product1 : Product  OutDataTypeStr=Inherit: Same as first input
  Product2 : Product  OutDataTypeStr=Inherit: Same as first input
  Real-Imag to Complex : RealImagToComplex
  Real-Imag to Complex1 : RealImagToComplex
  Sum3 : Sum  Inputs=|++  OutDataTypeStr=Inherit: Same as first input
  Sum4 : Sum  Inputs=|+-  OutDataTypeStr=Inherit: Inherit via back propagation
  Sum5 : Sum  Inputs=|++  OutDataTypeStr=Inherit: Same as first input
  Sum6 : Sum  Inputs=|++  OutDataTypeStr=Inherit: Same as first input
  Switch : Switch  Criteria=u2 ~= 0  OutDataTypeStr=Inherit: Inherit via back propagation
  Switch1 : Switch  Criteria=u2 ~= 0  OutDataTypeStr=Inherit: Inherit via back propagation
  Switch6 : Switch  Criteria=u2 ~= 0  OutDataTypeStr=Inherit: Inherit via back propagation
  atan2 : helperLib/atan2
      link override inv Lookup Table: OutDataTypeStr=fixdt(1,16,2)  BreakpointsForDimension1=-16:frac_lut_res_cr:15  Table=[(1./(-16:frac_lut_res_cr:(0-frac_lut_res_cr))), 1/frac_lut_res_cr, (1./((0+frac_lut_res_cr):frac_lut_res_cr:15))]  RemoveProtectionInput=off
  complex_magnitude_sq : helperLib/complex_magnitude_sq
  cr_pre_amp : Gain  Gain=cr_pre_amp  OutDataTypeStr=Inherit: Same as input
  find_nearest : Subsystem
  mult_delay{,1..6} (7 alike) : Delay  DelayLength=mult_pipeline
  mult_delay_match : Delay  DelayLength=mult_pipeline
  mult_delay_match1 : Delay  DelayLength=mult_pipeline*4+regular_pipeline*2
  mult_delay_match2 : Delay  DelayLength=mult_pipeline
  pipeline_delay{2..5,7} (5 alike) : Delay  DelayLength=regular_pipeline
  Recovered Const I : Outport  PortDimensions=1  SampleTime=overSamplePer
  Recovered Const Q : Outport  Port=2  PortDimensions=1  SampleTime=overSamplePer
  Phase Offset : Outport  Port=3  PortDimensions=1  SampleTime=overSamplePer
  After Loop Filter : Outport  Port=4  PortDimensions=1  SampleTime=overSamplePer
  Cumulative : Outport  Port=5  PortDimensions=1  SampleTime=overSamplePer
  wires:
  I/1 -> Real-Imag to Complex/1
  Q/1 -> Real-Imag to Complex/2
  Complex to Real-Imag/2 -> Gain/1
  Gain/1 -> mult_delay5/1
  Complex to Real-Imag/1 -> mult_delay_match/1
  Product/1 -> mult_delay1/1
  Product1/1 -> mult_delay/1
  1-D Lookup Table/1 -> mult_delay2/1
  Complex to Real-Imag2/1 -> Recovered Const I/1
  Complex to Real-Imag2/2 -> Recovered Const Q/1
  Sum4/1 -> pipeline_delay5/1
  Compare To Constant3/1 -> Switch/2
  Compare To Constant2/1 -> Switch1/2
  Constant1/1 -> Switch/1, Switch1/1
  Constant2/1 -> Switch1/3, Switch/3
  Switch/1 -> Sum5/2
  Sum5/1 -> Sum4/1
  Switch1/1 -> Sum4/2
  Shift180/1 -> Switch6/2
  Constant9/1 -> Switch6/1
  Constant8/1 -> Switch6/3
  Sum6/1 -> pipeline_delay4/1
  Switch6/1 -> Sum6/2
  Loop Filter/1(Out1) -> Sum6/1, After Loop Filter/1
  Sum3/1 -> Sum5/1, Compare To Constant3/1, Compare To Constant2/1
  pipeline_delay4/1 -> Sum3/1
  pipeline_delay5/1 -> Sum3/2, mult_delay6/1, Cumulative/1
  mult_delay2/1 -> Product1/2
  mult_delay4/1 -> cr_pre_amp/1
  mult_delay_match2/1 -> Product/1
  Real-Imag to Complex1/1 -> Product/2
  mult_delay/1 -> mult_delay_match1/1, Complex to Real-Imag2/1, Data Type Conversion1/1
  Product2/1 -> mult_delay4/1
  mult_delay_match1/1 -> complex_magnitude_sq/1
  complex_magnitude_sq/1 -> pipeline_delay3/1
  mult_delay1/1 -> Complex to Real-Imag1/1
  cr_pre_amp/1 -> pipeline_delay7/1
  find_nearest/1(Out1) -> mult_delay_match2/1
  pipeline_delay7/1 -> Loop Filter/1(In1)
  Data Type Conversion1/1 -> find_nearest/1(In1), Complex to Real-Imag/1
  atan2/1 -> pipeline_delay2/1
  Complex to Real-Imag1/2 -> atan2/1
  Complex to Real-Imag1/1 -> atan2/2
  Data Type Conversion2/1 -> Product2/1, Phase Offset/1
  Real-Imag to Complex/1 -> mult_delay3/1
  mult_delay3/1 -> Product1/1
  pipeline_delay2/1 -> Data Type Conversion2/1
  pipeline_delay3/1 -> Product2/2
  mult_delay5/1 -> Real-Imag to Complex1/2
  mult_delay_match/1 -> Real-Imag to Complex1/1
  mult_delay6/1 -> 1-D Lookup Table/1

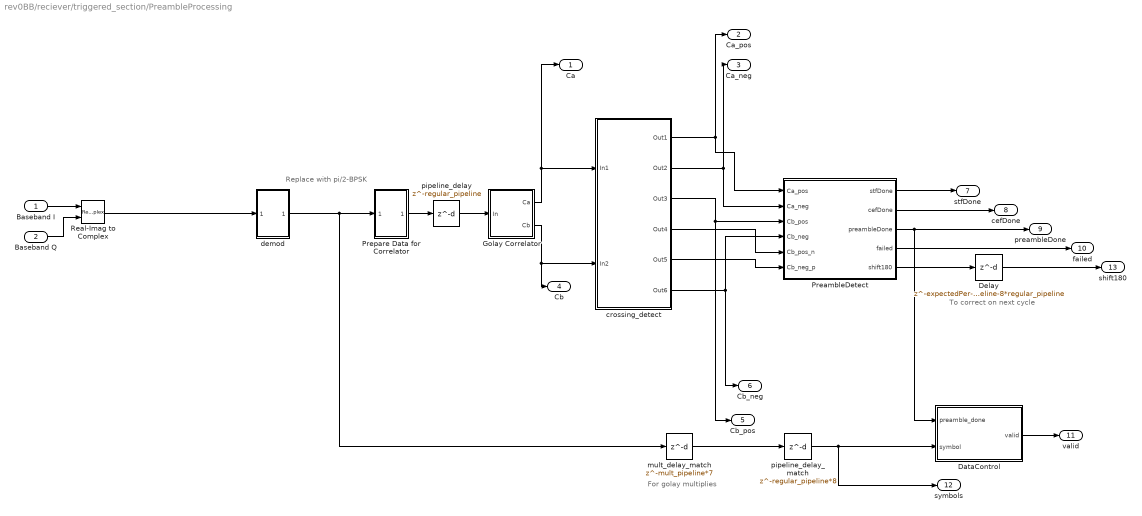
== system rev0BB/reciever/triggered_section/PreambleProcessing ==
  note: To correct on next cycle
  note: For golay multiplies
  note: Replace with pi/2-BPSK
  Baseband I : Inport  OutDataTypeStr=fixdt(1,14,11)
  Baseband Q : Inport  Port=2  OutDataTypeStr=fixdt(1,14,11)
  DataControl : Stateflow chart  TreatAsAtomicUnit=on
  Delay : Delay  DelayLength=expectedPer-7*mult_pipeline-8*regular_pipeline  InitialCondition=0
  Golay Correlator : Subsystem
  PreambleDetect : Stateflow chart  TreatAsAtomicUnit=on
  Prepare Data for Correlator : Subsystem
  Real-Imag to Complex : RealImagToComplex
  crossing_detect : Subsystem
  demod : Subsystem
  mult_delay_match : Delay  DelayLength=mult_pipeline*7
  pipeline_delay : Delay  DelayLength=regular_pipeline
  pipeline_delay_match : Delay  DelayLength=regular_pipeline*8
  Ca : Outport
  Ca_pos : Outport  Port=2  OutDataTypeStr=boolean
  Ca_neg : Outport  Port=3  OutDataTypeStr=boolean
  Cb : Outport  Port=4
  Cb_pos : Outport  Port=5  OutDataTypeStr=boolean
  Cb_neg : Outport  Port=6  OutDataTypeStr=boolean
  stfDone : Outport  Port=7
  cefDone : Outport  Port=8
  preambleDone : Outport  Port=9
  failed : Outport  Port=10
  valid : Outport  Port=11
  symbols : Outport  Port=12
  shift180 : Outport  Port=13
  wires:
  Prepare Data for Correlator/1(Out1) -> pipeline_delay/1
  PreambleDetect/3(preambleDone) -> DataControl/1(preamble_done), preambleDone/1
  Baseband I/1 -> Real-Imag to Complex/1
  Baseband Q/1 -> Real-Imag to Complex/2
  DataControl/1(valid) -> valid/1
  PreambleDetect/2(cefDone) -> cefDone/1
  Golay Correlator/1(Ca) -> Ca/1, crossing_detect/1(In1)
  PreambleDetect/4(failed) -> failed/1
  PreambleDetect/5(shift180) -> Delay/1
  Golay Correlator/2(Cb) -> crossing_detect/2(In2), Cb/1
  PreambleDetect/1(stfDone) -> stfDone/1
  pipeline_delay/1 -> Golay Correlator/1(In)
  pipeline_delay_match/1 -> DataControl/2(symbol), symbols/1
  mult_delay_match/1 -> pipeline_delay_match/1
  Delay/1 -> shift180/1
  demod/1(Out1) -> mult_delay_match/1, Prepare Data for Correlator/1(In1)
  Real-Imag to Complex/1 -> demod/1(In1)
  crossing_detect/3(Out3) -> Cb_pos/1, PreambleDetect/3(Cb_pos)
  crossing_detect/2(Out2) -> PreambleDetect/2(Ca_neg), Ca_neg/1
  crossing_detect/6(Out6) -> Cb_neg/1, PreambleDetect/4(Cb_neg)
  crossing_detect/1(Out1) -> PreambleDetect/1(Ca_pos), Ca_pos/1
  crossing_detect/4(Out4) -> PreambleDetect/5(Cb_pos_n)
  crossing_detect/5(Out5) -> PreambleDetect/6(Cb_neg_p)

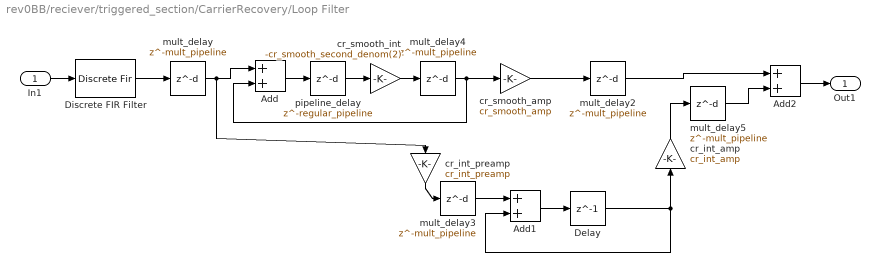
== system rev0BB/reciever/triggered_section/CarrierRecovery/Loop Filter ==
  In1 : Inport
  Add : Sum
  Add1 : Sum
  Add2 : Sum
  Delay : Delay  DelayLength=1  InitialCondition=0
  Discrete FIR Filter : DiscreteFir  FilterStructure=Direct form symmetric  Coefficients=cr_smooth_num  OutDataTypeStr=Inherit: Same as input
  cr_int_amp : Gain  Gain=cr_int_amp  OutDataTypeStr=Inherit: Same as input
  cr_int_preamp : Gain  Gain=cr_int_preamp  OutDataTypeStr=Inherit: Same as input
  cr_smooth_amp : Gain  Gain=cr_smooth_amp  OutDataTypeStr=Inherit: Same as input
  cr_smooth_int : Gain  Gain=-cr_smooth_second_denom(2)  OutDataTypeStr=Inherit: Same as input
  mult_delay{,2..5} (5 alike) : Delay  DelayLength=mult_pipeline
  pipeline_delay : Delay  DelayLength=regular_pipeline
  Out1 : Outport
  wires:
  cr_smooth_amp/1 -> mult_delay2/1
  In1/1 -> Discrete FIR Filter/1
  Discrete FIR Filter/1 -> mult_delay/1
  Add/1 -> pipeline_delay/1
  mult_delay2/1 -> Add2/1
  cr_smooth_int/1 -> mult_delay4/1
  mult_delay/1 -> cr_int_preamp/1, Add/1
  Add1/1 -> Delay/1
  mult_delay4/1 -> cr_smooth_amp/1, Add/2
  cr_int_preamp/1 -> mult_delay3/1
  cr_int_amp/1 -> mult_delay5/1
  mult_delay3/1 -> Add1/1
  Add2/1 -> Out1/1
  mult_delay5/1 -> Add2/2
  Delay/1 -> Add1/2, cr_int_amp/1
  pipeline_delay/1 -> cr_smooth_int/1

== system rev0BB/reciever/triggered_section/CarrierRecovery/find_nearest ==
  In1 : Inport
  BPSK Demodulator Baseband : commdigbbndpm3/BPSK Demodulator Baseband  Ph=0  DecType=Hard decision  VarSource=Dialog  Variance=1  outDtype=boolean  derotateFactorWordLen=16
  BPSK Modulator Baseband : commdigbbndpm3/BPSK Modulator Baseband  Ph=0  outDtype=Fixed-point  outWordLen=16  outUDDataType=sfix(16)  outFracLenMode=User-defined  outFracLen=11
  Out1 : Outport
  wires:
  BPSK Modulator Baseband/1 -> Out1/1
  BPSK Demodulator Baseband/1 -> BPSK Modulator Baseband/1
  In1/1 -> BPSK Demodulator Baseband/1

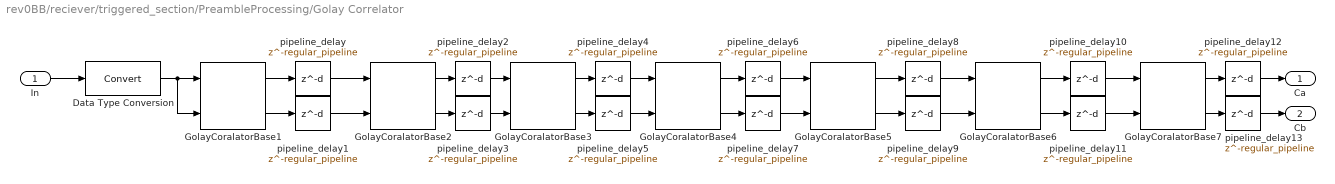
== system rev0BB/reciever/triggered_section/PreambleProcessing/Golay Correlator ==
  In : Inport
  Data Type Conversion : DataTypeConversion
  GolayCoralatorBase1 : golayLib/GolayCoralatorBase  dSub=D_128(1)  wSub=W_128(1)
  GolayCoralatorBase2 : golayLib/GolayCoralatorBase  dSub=D_128(2)  wSub=W_128(2)
  GolayCoralatorBase3 : golayLib/GolayCoralatorBase  dSub=D_128(3)  wSub=W_128(3)
  GolayCoralatorBase4 : golayLib/GolayCoralatorBase  dSub=D_128(4)  wSub=W_128(4)
  GolayCoralatorBase5 : golayLib/GolayCoralatorBase  dSub=D_128(5)  wSub=W_128(5)
  GolayCoralatorBase6 : golayLib/GolayCoralatorBase  dSub=D_128(6)  wSub=W_128(6)
  GolayCoralatorBase7 : golayLib/GolayCoralatorBase  dSub=D_128(7)  wSub=W_128(7)
  pipeline_delay{,1..13} (14 alike) : Delay  DelayLength=regular_pipeline
  Ca : Outport
  Cb : Outport  Port=2
  wires:
  GolayCoralatorBase1/1 -> pipeline_delay/1
  GolayCoralatorBase1/2 -> pipeline_delay1/1
  GolayCoralatorBase2/1 -> pipeline_delay2/1
  GolayCoralatorBase2/2 -> pipeline_delay3/1
  GolayCoralatorBase5/1 -> pipeline_delay8/1
  GolayCoralatorBase3/1 -> pipeline_delay4/1
  GolayCoralatorBase3/2 -> pipeline_delay5/1
  GolayCoralatorBase4/1 -> pipeline_delay6/1
  GolayCoralatorBase4/2 -> pipeline_delay7/1
  GolayCoralatorBase5/2 -> pipeline_delay9/1
  GolayCoralatorBase6/2 -> pipeline_delay11/1
  GolayCoralatorBase6/1 -> pipeline_delay10/1
  GolayCoralatorBase7/2 -> pipeline_delay13/1
  GolayCoralatorBase7/1 -> pipeline_delay12/1
  In/1 -> Data Type Conversion/1
  Data Type Conversion/1 -> GolayCoralatorBase1/2, GolayCoralatorBase1/1
  pipeline_delay/1 -> GolayCoralatorBase2/1
  pipeline_delay1/1 -> GolayCoralatorBase2/2
  pipeline_delay2/1 -> GolayCoralatorBase3/1
  pipeline_delay3/1 -> GolayCoralatorBase3/2
  pipeline_delay4/1 -> GolayCoralatorBase4/1
  pipeline_delay5/1 -> GolayCoralatorBase4/2
  pipeline_delay6/1 -> GolayCoralatorBase5/1
  pipeline_delay7/1 -> GolayCoralatorBase5/2
  pipeline_delay8/1 -> GolayCoralatorBase6/1
  pipeline_delay9/1 -> GolayCoralatorBase6/2
  pipeline_delay10/1 -> GolayCoralatorBase7/1
  pipeline_delay11/1 -> GolayCoralatorBase7/2
  pipeline_delay12/1 -> Ca/1
  pipeline_delay13/1 -> Cb/1

== system rev0BB/reciever/triggered_section/PreambleProcessing/Prepare Data for Correlator ==
  In1 : Inport  OutDataTypeStr=uint8
  Add1 : Sum  Inputs=+-  OutDataTypeStr=fixdt(1,8,0)
  Bit Shift : hdlsllib/HDL Operations/Bit Shift  mode=Shift Left Logical  N=1
  Constant3 : Constant  OutDataTypeStr=fixdt(1,8,0)
  Out1 : Outport  OutDataTypeStr=int8
  wires:
  Constant3/1 -> Add1/2
  Bit Shift/1 -> Add1/1
  Add1/1 -> Out1/1
  In1/1 -> Bit Shift/1

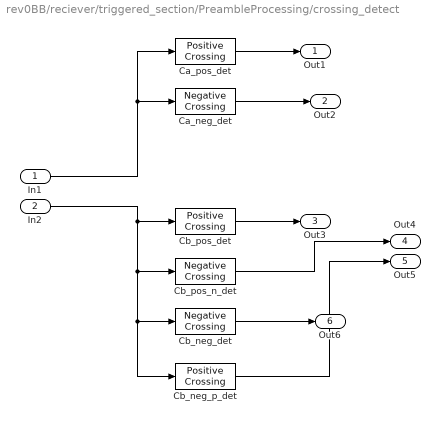
== system rev0BB/reciever/triggered_section/PreambleProcessing/crossing_detect ==
  In1 : Inport
  In2 : Inport  Port=2
  Ca_neg_det : helperLib/Negative Crossing  crossPt=-trigger
  Ca_pos_det : helperLib/Positive Crossing  crossPt=trigger
  Cb_neg_det : helperLib/Negative Crossing  crossPt=-trigger
  Cb_neg_p_det : helperLib/Positive Crossing  crossPt=-trigger
  Cb_pos_det : helperLib/Positive Crossing  crossPt=trigger
  Cb_pos_n_det : helperLib/Negative Crossing  crossPt=trigger
  Out1 : Outport
  Out2 : Outport  Port=2
  Out3 : Outport  Port=3
  Out4 : Outport  Port=4
  Out5 : Outport  Port=5
  Out6 : Outport  Port=6
  wires:
  In1/1 -> Ca_pos_det/1, Ca_neg_det/1
  Cb_neg_p_det/1 -> Out5/1
  Cb_pos_n_det/1 -> Out4/1
  Cb_pos_det/1 -> Out3/1
  Ca_pos_det/1 -> Out1/1
  Cb_neg_det/1 -> Out6/1
  Ca_neg_det/1 -> Out2/1
  In2/1 -> Cb_neg_p_det/1, Cb_neg_det/1, Cb_pos_n_det/1, Cb_pos_det/1

== system rev0BB/reciever/triggered_section/PreambleProcessing/demod ==
  In1 : Inport
  BPSK Demodulator Baseband : commdigbbndpm3/BPSK Demodulator Baseband  Ph=0  DecType=Hard decision  VarSource=Dialog  Variance=1  outDtype=uint8  derotateFactorWordLen=16
  Out1 : Outport
  wires:
  BPSK Demodulator Baseband/1 -> Out1/1
  In1/1 -> BPSK Demodulator Baseband/1

== stateflow chart rev0BB/reciever/triggered_section/PreambleProcessing/DataControl ==
  settings: executeAtInitialization=1
  note: Start Symbol is a series of 8 1's (del char)
  state Search_for_start
    entry:
    startCount = startCount + int32(1);
    waitCount = waitCount + int32(1);
  state Data
    entry:
    valid = true;
    dataCount = dataCount + int32(1);
  state Waiting
    entry:
    valid = false;
    startCount = int32(0);
    dataCount = int32(0);
    waitCount = int32(0);
  Data -> Data [order 2]
  (default) -> Waiting
  Search_for_start -> Search_for_start [order 3] : [symbol == 1 && startCount <= 8]
  Search_for_start -> Data [order 1] : [startCount > 8]
  Waiting -> Search_for_start : [preamble_done == true]
  Data -> Waiting [order 1] : [dataCount >= dataLen]
  Search_for_start -> Waiting [order 2] : [waitCount > guardInt+guardTol+wordLen]
  Search_for_start -> Search_for_start [order 4] : [symbol == 0]/{startCount = int32(0);}
  data: preamble_done input boolean; symbol input; valid output boolean; startCount local int32; dataCount local int32; buffer local boolean size=8; guardInt parameter int32; guardTol parameter int32; waitCount local int32; wordLen parameter int32; dataLen parameter int32

== matlab function rev0BB/MATLAB Function ==
  data: symbolIn input; valid input; lineWidth input
function decodeText(symbolIn,valid,lineWidth)
%DECODE_TEXT Decodes text as it is recieved
persistent count;
persistent lineCount;
persistent symbolBuffer;
persistent prevValid;

if isempty(prevValid)
    prevValid = false;
end
    
if isempty(count)
    count = 0;
end

if isempty(symbolBuffer)
    symbolBuffer = 0;
end

if isempty(lineCount)
    lineCount = 0;
end

if(valid)
    %Buffer the newest symbol (binary)
    newBit = 0;
    if(symbolIn ~= 0 )
        newBit = 1;
    end

    symbolBuffer = symbolBuffer * 2;
    symbolBuffer = symbolBuffer + newBit;
    count = count+1;

    %%have full char, now decode and reset
    if(count >= 8)
        if(symbolBuffer <= 2^7)
            newChar = char(symbolBuffer);
        else
            newChar = '$';
        end
        fprintf('%s', newChar);
        count = 0;
        symbolBuffer = 0;
        lineCount = lineCount+1;
        if(lineCount>lineWidth && newChar==' ')
            fprintf('\n');
            lineCount = 0;
        end
    end
%else
%    count = 0;
%    symbolBuffer = 0;
end

== stateflow chart rev0BB/reciever/triggered_section/PreambleProcessing/PreambleDetect ==
  settings: executeAtInitialization=1
  note: Need to hold done for 5 cycles (due to rate conversion)
  state Waiting
    entry:
    stfDone = false;
    cefDone = false;
    preambleDone = false;
    shift180 = false;
    failed = false;
  state STF
    state STF_Neg
      entry:
      cbCount = cbCount + int32(1);
      counter = int32(1);
      during:
      counter = counter +int32(1);
    state STF_Initial_Correct
      during:
      counter = counter +int32(1);
    state STF_WaitNegEdge
      entry:
      during:
      counter = counter +int32(1);
    state STF_Transitioning_WaitNegEdge
      entry:
      during:
      counter = counter +int32(1);
    state STF_Transitioning_Inverted
      entry:
      cbCount = cbCount + int32(1);
      counter = int32(1);
      during:
      counter = counter +int32(1);
    state STF_Initial_Inverted
      entry:
      cbCount = cbCount + int32(1);
      counter = int32(1);
      during:
      counter = counter +int32(1);
    state STF_Inverted_WaitNegEdge
      entry:
      during:
      counter = counter +int32(1);
    state CorrectPhase
      entry:
      cbCount = cbCount + int32(1);
      counter = int32(1);
      shift180 = true;
      during:
      counter = counter +int32(1);
    STF_WaitNegEdge -> STF_Initial_Correct [order 1] : [Cb_pos_n == 1]/
        | {
        |  cbCount = cbCount + 1;
        |  counter = int32(1);}
    STF_Initial_Correct -> STF_WaitNegEdge [order 3] : [Cb_pos == 1]
    STF_Initial_Correct -> STF_Neg [order 5] : [Cb_neg == 1]
    STF_Transitioning_WaitNegEdge -> STF_Initial_Correct [order 1] : [Cb_neg_p == 1]/
        | { counter = int32(1);}
    STF_Transitioning_Inverted -> STF_Transitioning_WaitNegEdge [order 1] : [Cb_neg == 1]
    STF_Transitioning_WaitNegEdge -> STF_Transitioning_Inverted [order 3] : [Cb_neg_p == 1]/
        | {}
    CorrectPhase -> STF_Transitioning_Inverted : {shift180 = false;}
    STF_Inverted_WaitNegEdge -> STF_Initial_Inverted [order 2] : [Cb_neg_p == 1]/
        | {}
    STF_Inverted_WaitNegEdge -> CorrectPhase [order 1] : [Cb_neg_p == 1 && cbCount > invertedTol]/
        | {}
    STF_Initial_Inverted -> STF_Inverted_WaitNegEdge [order 1] : [Cb_neg == 1]
  state CEF
    note: Need actual logic for CEF, right now only checks for correct sequence
    state STF_Done
      entry:
      stfDone = true;
      cbCount = cbCount + int32(1);
      counter = int32(1);
      during:
      counter = counter +int32(1);
    state CEF_Checking
      entry:
      cefCount = cefCount + int32(1);
      counter = int32(1);
      during:
      counter = counter +int32(1);
    STF_Done -> CEF_Checking [order 3] : [Cb_neg == 1]/{
        | cefCount = int32(1);
        | }
  state Failed
    entry:
    failed = true;
  state Done
    entry:
    cefDone = true;
    preambleDone = true;
    counter = int32(0);
    during:
    counter = counter + int32(1);
  CEF_Checking -> Failed [order 4] : [cefSeqCheck(Ca_pos,Ca_neg,Cb_pos, Cb_neg, cefCount) == 1 && counter <(expectedPer-tol)]
  STF_Done -> Failed [order 2] : [Cb_neg == 1 && counter <(expectedPer-tol)]
  STF_Neg -> Failed [order 2] : [Ca_neg == 1 && counter <(expectedPer-tol)]
  STF_Neg -> Failed [order 1] : [Cb_neg == 1 || Ca_pos == 1 || Cb_pos == 1  || counter >(expectedPer+tol)]
  STF_WaitNegEdge -> Failed [order 2] : [counter > expectedPer+tol]
  Done -> Waiting : [counter > 4]
  (default) -> Waiting
  Failed -> Waiting
  STF_Initial_Correct -> Waiting [order 1] : [Cb_pos == 1 && counter <(expectedPer-tol)]
  CEF_Checking -> CEF_Checking [order 2] : [cefSeqCheck(Ca_pos,Ca_neg,Cb_pos, Cb_neg, cefCount) == 1 && cefCount < cef_note_len]
  CEF_Checking -> Failed [order 1] : [cefSeqCheck(Ca_pos,Ca_neg,Cb_pos, Cb_neg, cefCount) == 0 || counter >(expectedPer+tol) || cefCount > cef_note_len]
  STF_Initial_Inverted -> Failed [order 2] : [Ca_pos ==  1 || Ca_neg == 1 || counter >(expectedPer+tol) || cbCount > 48 + cbTol]
  STF_Done -> Failed [order 1] : [Ca_pos == 1 || Ca_neg == 1 || Cb_pos == 1 || counter >(128+expectedPer)]
  STF_Initial_Correct -> Failed [order 4] : [Ca_pos ==  1 || Ca_neg == 1 || counter >(expectedPer+tol) || cbCount > 48 + cbTol]
  STF_Inverted_WaitNegEdge -> Failed [order 3] : [counter > expectedPer+tol]
  STF_Initial_Correct -> Failed [order 2] : [Cb_neg && (cbCount < 48 - cbTol)]
  STF_Transitioning_Inverted -> Failed [order 2] : [counter > expectedPer+tol]
  STF_Transitioning_WaitNegEdge -> Failed [order 2] : [counter > expectedPer+tol]
  Waiting -> STF_Initial_Inverted [order 2] : [Cb_neg == 1]/
      | {
      | cbCount = int32(0);
      | counter = expectedPer;
      | }
  Waiting -> STF_Initial_Correct [order 1] : [Cb_pos == 1]/
      | {
      | cbCount = int32(0);
      | counter = int32(1);
      | }
  STF_Neg -> STF_Done [order 3] : [Ca_neg == 1]
  CEF_Checking -> Done [order 3] : [cefSeqCheck(Ca_pos,Ca_neg,Cb_pos, Cb_neg, cefCount) == 1 && cefCount == cef_note_len]
  data: Ca_p function_input; Ca_n function_input; Cb_p function_input; Cb_n function_input; cnt function_input; ok function_output boolean; Ca_pos input boolean; Ca_neg input boolean; tol parameter int32; Cb_pos input boolean; Cb_neg input boolean; cbTol parameter int32; counter local int32; cbCount local int32; stfDone output boolean; cef_note_len parameter uint16; cefDone output boolean; preambleDone output boolean; cefCount local int32; failed output boolean; expectedPer parameter int32; expectedWidth parameter int32; Cb_pos_n input boolean; Cb_neg_p input boolean; invertedTol parameter int32; shift180 output boolean
  function ok = cefSeqCheck(Ca_p, Ca_n, Cb_p, Cb_n, cnt):
    | function ok = cefSeqCheck(Ca_p, Ca_n, Cb_p, Cb_n, cnt)
    | % cannot pass in array as parameter unfortuantly
    | Gu_512_note = [-2, -1, 2, -1];
    | Gv_512_note = [-2, 1, -2, -1];
    | Gv_128_note = Gv_512_note(1);
    | cef_note  = cat(2, Gu_512_note, Gv_512_note, Gv_128_note);
    | cef_note  = int16(cef_note);
    | 
    | if(Ca_p == 0 && Ca_n == 0 && Cb_p == 0 && Cb_n == 0)
    |     ok = 2; %% not triggered
    | else
    |     switch(cef_note(cnt))
    |         case 1
    |             if(Ca_p == 1)
    |                 ok = 1;
    |             else
    |                 ok = 0;
    |             end
    |         case 2
    |             if(Cb_p == 1)
    |                 ok = 1;
    |             else
    |                 ok = 0;
    |             end
    |         case -1
    |             if(Ca_n == 1)
    |                 ok = 1;
    |             else
    |                 ok = 0;
    |             end
    |         case -2
    |             if(Cb_n == 1)
    |                 ok = 1;
    |             else
    |                 ok = 0;
    |             end
    |         otherwise
    |             ok = 0;
    |     end
    | end
    | end
